simulink model "MPC_proper_simulation"  (R2020b)
settings: Solver=ode15s  StartTime=0.0  StopTime=100  RelTol=1e-3
settings Model: Creator=surya  LastModifiedBy=surya

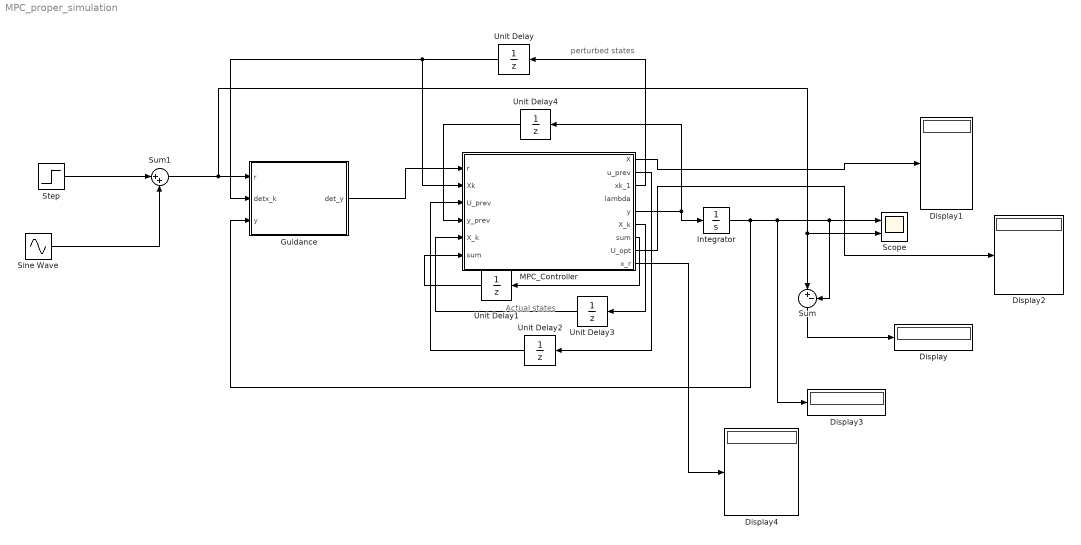
== system MPC_proper_simulation ==
  note: Actual states
  note: perturbed states
  Display{,1..4} (5 alike) : Display
  Guidance : MATLAB Function  TreatAsAtomicUnit=on
  Integrator : Integrator
  MPC_Controller : MATLAB Function  TreatAsAtomicUnit=on
  Scope : Scope  NumInputPorts=2
  Sine Wave : Sin  SampleTime=0
  Step : Step  After=50  SampleTime=0
  Sum : Sum  Inputs=|+-
  Sum1 : Sum  Inputs=|++
  Unit Delay : UnitDelay  InitialCondition=[0 0 0 0]  SampleTime=-1  HasFrameUpgradeWarning=on
  Unit Delay1 : UnitDelay  SampleTime=-1  HasFrameUpgradeWarning=on
  Unit Delay2 : UnitDelay  SampleTime=-1  HasFrameUpgradeWarning=on
  Unit Delay3 : UnitDelay  InitialCondition=[15 0.0393 0 0.0393]  SampleTime=-1  HasFrameUpgradeWarning=on
  Unit Delay4 : UnitDelay  SampleTime=-1  HasFrameUpgradeWarning=on
  wires:
  Guidance/1(det_y) -> MPC_Controller/1(r)
  MPC_Controller/5(y) -> Integrator/1, Unit Delay4/1
  Integrator/1 -> Guidance/3(y), Display3/1, Sum/2, Scope/1
  MPC_Controller/3(xk_1) -> Unit Delay/1
  Unit Delay/1 -> MPC_Controller/2(Xk), Guidance/2(detx_k)
  MPC_Controller/7(sum) -> Unit Delay1/1
  Unit Delay1/1 -> MPC_Controller/6("sum ")
  MPC_Controller/6(X_k) -> Unit Delay3/1
  Unit Delay3/1 -> MPC_Controller/5("X_k ")
  MPC_Controller/2(u_prev) -> Unit Delay2/1
  Unit Delay2/1 -> MPC_Controller/3(U_prev)
  Sum/1 -> Display/1
  Sine Wave/1 -> Sum1/2
  Sum1/1 -> Scope/2, Sum/1, Guidance/1(r)
  Step/1 -> Sum1/1
  Unit Delay4/1 -> MPC_Controller/4(y_prev)
  MPC_Controller/8(U_opt) -> Display2/1
  MPC_Controller/1(X) -> Display1/1
  MPC_Controller/9(x_r) -> Display4/1

== matlab function MPC_proper_simulation/MPC_Controller ==
  data: X output; u_prev output; xk_1 output; lambda output; r input; y output; X_k output; Xk input; U_prev input; y_prev input; X_k input; sum input; sum output; U_opt output; x_r output
function [X,u_prev,xk_1,lambda,y,X_k,sum,U_opt,x_r] = MPC_Controller(r, Xk, U_prev, y_prev, X_k, sum)

N = 5;

xk = Xk;  %Perturbed states used in State Space
det_t = 0.1;

A = [-1.9311*10^-2 8.8157 -32.17 -0.575; -2.5389*10^-4 -1.0189 0 0.9051; 2.9465*10^-12 0.8223 0 -1.0774; 0 0 1 0];
B = [0.1737; -2.1499; -0.1756; 0];
C = [(sin(X_k(4))-(tan(X_k(2))*cos(X_k(4)))) -X_k(1)*cos(X_k(4))*(sec(X_k(2)))^2 0 X_k(1)*(cos(X_k(4))+(tan(X_k(2))*sin(X_k(4))))]*det_t;  %Change C, because Jacobian should be taken wrt to [det_u, det_alpha, det_q, det_theta] and not [u, alpha, q, theta]
D = 0;

fx = [sign(xk(1)) 0 0 0; 0 sign(xk(2)) 0 0; 0 0 sign(xk(3)) 0; 0 0 0 sign(xk(4))];
Fx = [fx, zeros([4,4]), zeros([4,4]), zeros([4,4]), zeros([4,4]); zeros([4,4]), fx, zeros([4,4]), zeros([4,4]), zeros([4,4]); zeros([4,4]), zeros([4,4]), fx, zeros([4,4]), zeros([4,4]); zeros([4,4]), zeros([4,4]), zeros([4,4]), fx, zeros([4,4]); zeros([4,4]), zeros([4,4]), zeros([4,4]), zeros([4,4]), fx];
Fu = sign(U_prev)*eye(N);   % 8 deg max elevator deflection
bbx = [10*sign(xk(1));0.174*sign(xk(2));0.174*sign(xk(3));0.174*sign(xk(4))];
bx = [bbx;bbx;bbx;bbx;bbx];
bu = 0.174*ones([N,1])*sign(U_prev);

ref = inv([(A-eye(length(A))) B; C D])*[zeros([length(A),1]);r];
x_r = ref(1:4);
if abs(x_r(1))>10
    x_r(1) = sign(x_r(1))*10;
end
if abs(x_r(2))>0.174
    x_r(2) = sign(x_r(2))*0.174;
end
if abs(x_r(3))>0.174
    x_r(3) = sign(x_r(3))*0.174;
end
if abs(x_r(4))>0.174
    x_r(4) = sign(x_r(4))*0.174;
end
    
u_r = ref(5);
if abs(u_r)>0.174
    u_r = sign(u_r)*0.174;
end

xr = [x_r;x_r;x_r;x_r;x_r];
ur = u_r*ones([N,1]);

A_c = [A;A^2;A^3;A^4;A^5];
B_c = [B zeros([4,1]) zeros([4,1]) zeros([4,1]) zeros([4,1]); A*B B zeros([4,1]) zeros([4,1]) zeros([4,1]); A^2*B A*B B zeros([4,1]) zeros([4,1]); A^3*B A^2*B A*B B zeros([4,1]); A^4*B A^3*B A^2*B A*B B];

Q = [5*10^1 0 0 0; 0 5*10^1 0 0; 0 0 5*10^1 0; 0 0 0 5*10^1];   %2  3.768*10^2
R = 3.3311*10^2;   %4
P = [5*10^1 0 0 0; 0 5*10^1 0 0; 0 0 5*10^1 0; 0 0 0 5*10^1];   %2  3.768*10^2
Q_c = [Q zeros([4,4]) zeros([4,4]) zeros([4,4]) zeros([4,4]); zeros([4,4]) Q zeros([4,4]) zeros([4,4]) zeros([4,4]); zeros([4,4]) zeros([4,4]) Q zeros([4,4]) zeros([4,4]); zeros([4,4]) zeros([4,4]) zeros([4,4]) Q zeros([4,4]); zeros([4,4]) zeros([4,4]) zeros([4,4]) zeros([4,4]) P];
R_c = R*eye(N);
M = [Fu; Fx*B_c];
L = [bu; (bx-Fx*A_c*xk)];
J = -0.0135*10^-2;

lambda = -inv(eye(length(M*inv(B_c'*Q_c*B_c + R_c)*M')) + 0.5*M*inv(B_c'*Q_c*B_c + R_c)*M')*(M*inv(B_c'*Q_c*B_c + R_c)*(B_c'*Q_c*A_c*xk - B_c'*Q_c*xr - R_c'*ur) + L);
%lambda = -inv(0.5*M*inv(B_c'*Q_c*B_c + R_c)*M')*(M*inv(B_c'*Q_c*B_c + R_c)*(B_c'*Q_c*A_c*xk - B_c'*Q_c*xr - R_c'*ur) + L);
U_opt = -inv(B_c'*Q_c*B_c + R_c)*(B_c'*Q_c*A_c*xk - B_c'*Q_c*xr - R_c'*ur + 0.5*M'*lambda);

if abs(r) < 5*10^-1
    sum = sum + r;
    det_u = J*sum*ones([N,1]);
else
    det_u = zeros([N,1]);
end

U_prev = U_opt + det_u;

if abs(U_prev(1)) > 0.174
    U_prev(1) = sign(U_prev(1))*0.174;
end
if abs(U_prev(2)) > 0.174
    U_prev(2) = sign(U_prev(2))*0.174;
end
if abs(U_prev(3)) > 0.174
    U_prev(3) = sign(U_prev(3))*0.174;
end
if abs(U_prev(4)) > 0.174
    U_prev(4) = sign(U_prev(4))*0.174;
end
if abs(U_prev(5)) > 0.174
    U_prev(5) = sign(U_prev(5))*0.174;
end

X = A_c*xk + B_c*U_prev;
u_prev = U_prev(1);
% Constraints
%X = (X<inv(Fx)*bx).*X + (X>inv(Fx)*bx).*(inv(Fx)*bx);
% if Fx*X < bx
%     
% else
%    X = (X<inv(Fx)*bx).*X + (X>inv(Fx)*bx).*(inv(Fx)*bx); 
% end

%xk_1 = A*xk + B*u_prev;
xk_1 = X(1:4);
% Constraint
%xk_1 = (fx*xk_1<bbx).*xk_1 + (fx*xk_1>bbx).*(inv(fx)*bbx);

y = C*xk;
X_k = X_k + xk_1;

end

== matlab function MPC_proper_simulation/Guidance ==
  data: det_y output; r input; detx_k input; y input
function det_y  = fcn(r,detx_k,y)

det_y = (r-y)/1;
